simulink model "PRBS_Test"  (R2019a)
settings: Solver=FixedStepAuto  StartTime=0.0  StopTime=TSim  FixedStep=0.2  RelTol=1e-3
values from neighbouring files (symbols this model uses):
  AMtx = [-8.08083e-02, -1.00674e-01, -1.60269e-01, -2.19865e-01, -2.79461e-01, -3.39057e-01, -3.98653e-01, -4.58249e-01, -5.17844e-01, -5.77440e-01, -6.37036e-01, -6.96632e-01]    [Test.m]
  BMtx = [1.54238e+05, 1.56531e+05, 1.63413e+05, 1.70294e+05, 1.77175e+05, 1.84056e+05, 1.90937e+05, 1.97818e+05, 2.04700e+05, 2.11581e+05, 2.18462e+05, 2.25343e+05]    [Test.m]
  NCMtx = ones(1,length(AMtx))    [Test.m]
  NDMtx = 0 * ones(1,length(AMtx))    [Test.m]
  NMtx = 23042*[2.16995e-02, 4.33990e-02, 1.08498e-01, 1.73596e-01, 2.38695e-01, 3.03793e-01, 3.68892e-01, 4.33990e-01, 4.99089e-01, 5.64187e-01, 6.29286e-01, 6.94384e-01]    [Test.m]
  Num_Switch = 50    [MissionBlocks.m]    (also in Test.m = 1)
  Percent = 0.1    [MissionBlocks.m]    (also in Test.m)
  RPM = NMtx(2)    [Test.m]
  Samp_end = 2    [MissionBlocks.m]    (also in Test.m)
  Samp_start = 100    [MissionBlocks.m]    (also in Test.m)
  Samp_Switch = 2    [MissionBlocks.m]    (also in Test.m = 1000)
  Ts = 0.2    [MissionBlocks.m]    (also in Test.m)
  Wf = [0.01335 0.01669 0.02 0.025 0.03 0.0334 0.04172 0.05 0.05841 0.06676]    [MissionBlocks.m]    (also in Test.m = WfMtx(2))
  WfMtx = [3.35319e-03, 4.47091e-03, 7.87431e-03, 1.14579e-02, 1.66929e-02, 2.16627e-02, 2.55503e-02, 2.86499e-02, 3.21360e-02, 3.58686e-02, 4.06799e-02, 4.63335e-02]    [Test.m]
libraries: ctrlSharedLib x2
settings Model: Creator=anton  LastModifiedBy=anton

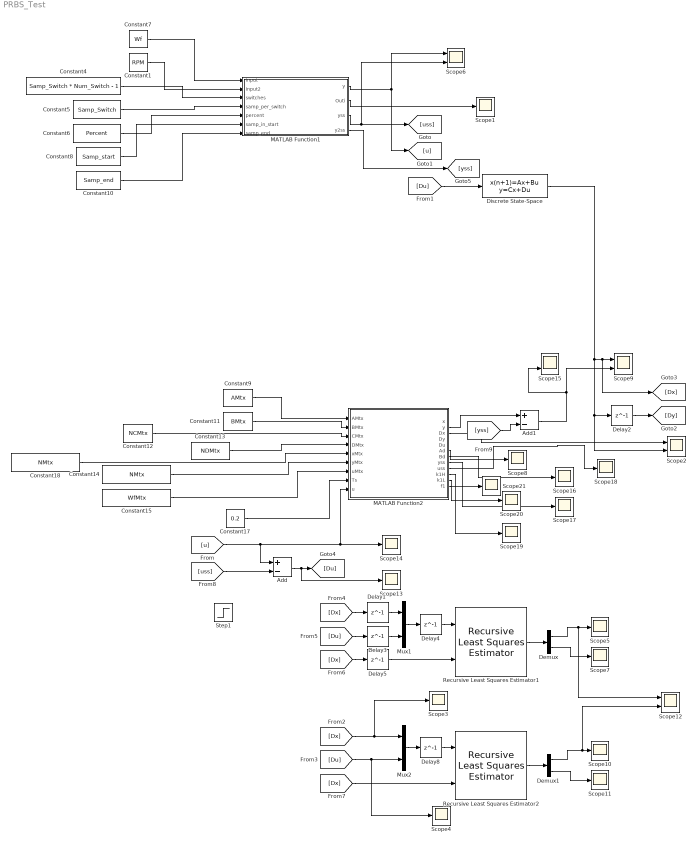
== system PRBS_Test ==
  Add : Sum  Inputs=+-
  Add1 : Sum  Inputs=+-
  Constant1 : Constant  Value=RPM
  Constant10 : Constant  Value=Samp_end
  Constant11 : Constant  Value=BMtx
  Constant12 : Constant  Value=NCMtx
  Constant13 : Constant  Value=NDMtx
  Constant14 : Constant  Value=NMtx
  Constant15 : Constant  Value=WfMtx
  Constant17 : Constant  Value=0.2
  Constant18 : Constant  Value=NMtx
  Constant4 : Constant  Value=Samp_Switch * Num_Switch - 1
  Constant5 : Constant  Value=Samp_Switch
  Constant6 : Constant  Value=Percent
  Constant7 : Constant  Value=Wf
  Constant8 : Constant  Value=Samp_start
  Constant9 : Constant  Value=AMtx
  Delay{1..5,8} (6 alike) : Delay  DelayLength=1  SampleTime=Ts
  Demux : Demux  Outputs=2
  Demux1 : Demux  Outputs=2
  Discrete State-Space : DiscreteStateSpace  A=0.9801  B=3.099e04  D=0  SampleTime=0.2
  MATLAB Function1 : MATLAB Function  TreatAsAtomicUnit=on
  MATLAB Function2 : MATLAB Function  TreatAsAtomicUnit=on
  Mux1 : Mux  Inputs=2
  Mux2 : Mux  Inputs=2
  Recursive Least Squares Estimator1 : ctrlSharedLib/Recursive Least Squares Estimator  InitialEstimateSource=None  InitialParameterData=2  P0=1e4  InitialRegressors=0  InitialOutputs=0  History=Infinite  WindowLength=200  EstimationMethod=Forgetting Factor  AdaptationParameter=0.5  HasTimeVaryingAdaptationParameter=off  NormalizationBias=eps  OutputError=off  OutputP=off  AddEnablePort=off  InputProcessing=Sample-based  Ts=Ts
      settings: SourceProductName=Control System Toolbox  SourceProductBaseCode=CT
  Recursive Least Squares Estimator2 : ctrlSharedLib/Recursive Least Squares Estimator  InitialEstimateSource=None  InitialParameterData=2  P0=1e4  InitialRegressors=0  InitialOutputs=0  History=Infinite  WindowLength=200  EstimationMethod=Forgetting Factor  AdaptationParameter=0.5  HasTimeVaryingAdaptationParameter=off  NormalizationBias=eps  OutputError=off  OutputP=off  AddEnablePort=off  InputProcessing=Sample-based  Ts=Ts
      settings: SourceProductName=Control System Toolbox  SourceProductBaseCode=CT
  Scope{1,3..5,7..8,10..11,13..14,16..21} (16 alike) : Scope
  Scope{2,6,9,12,15} (5 alike) : Scope  NumInputPorts=2
  Step1 : Step  Time=50  Before=1.5  After=2.7  SampleTime=0
  wires:
  Constant6/1 -> MATLAB Function1/5(percent)
  Constant5/1 -> MATLAB Function1/4(samp_per_switch)
  Constant4/1 -> MATLAB Function1/3(switches)
  MATLAB Function1/1(y) -> Scope6/1, [u]
  Constant7/1 -> MATLAB Function1/1(Input)
  Constant8/1 -> MATLAB Function1/6(samp_in_start)
  Constant10/1 -> MATLAB Function1/7(samp_end)
  Constant9/1 -> MATLAB Function2/1(AMtx)
  Constant11/1 -> MATLAB Function2/2(BMtx)
  Constant12/1 -> MATLAB Function2/3(CMtx)
  Constant13/1 -> MATLAB Function2/4(DMtx)
  Constant14/1 -> MATLAB Function2/6(yMtx)
  Constant15/1 -> MATLAB Function2/7(uMtx)
  [u] -> Add/1, Scope14/1, MATLAB Function2/9(u)
  Constant17/1 -> MATLAB Function2/8(Ts)
  Constant18/1 -> MATLAB Function2/5(xMtx)
  MATLAB Function2/3(Dx) -> Scope2/1
  Recursive Least Squares Estimator1/1 -> Demux/1
  Demux/1 -> Scope12/1, Scope5/1
  Demux/2 -> Scope7/1
  Mux1/1 -> Delay4/1
  [Dx] -> Delay1/1
  [Du] -> Delay3/1
  [Dx] -> Delay5/1
  MATLAB Function2/2(y) -> Add1/1
  [Du] -> Discrete State-Space/1
  MATLAB Function1/2(Outi) -> Scope1/1
  Delay1/1 -> Mux1/1
  Delay3/1 -> Mux1/2
  Delay4/1 -> Recursive Least Squares Estimator1/1
  Delay5/1 -> Recursive Least Squares Estimator1/2
  Delay2/1 -> [Dy]
  Discrete State-Space/1 -> Scope2/2, Delay2/1, [Dx], Scope9/1
  [Dx] -> Recursive Least Squares Estimator2/2
  Delay8/1 -> Recursive Least Squares Estimator2/1
  [Du] -> Scope4/1, Mux2/2
  [Dx] -> Scope3/1, Mux2/1
  Mux2/1 -> Delay8/1
  Demux1/2 -> Scope11/1
  Demux1/1 -> Scope12/2, Scope10/1
  Recursive Least Squares Estimator2/1 -> Demux1/1
  MATLAB Function1/3(yss) -> Scope6/2, [uss]
  Add/1 -> Scope13/1, [Du]
  [uss] -> Add/2
  Constant1/1 -> MATLAB Function1/2(Input2)
  MATLAB Function1/4(y2ss) -> [yss]
  [yss] -> Add1/2
  Add1/1 -> Scope15/2, Scope9/2
  MATLAB Function2/6(Ad) -> Scope8/1
  MATLAB Function2/7(Bd) -> Scope16/1
  MATLAB Function2/8(yss) -> Scope17/1
  MATLAB Function2/9(uss) -> Scope18/1
  MATLAB Function2/10(k1H) -> Scope19/1
  MATLAB Function2/11(k1L) -> Scope20/1
  MATLAB Function2/12(f1) -> Scope21/1

== matlab function PRBS_Test/MATLAB Function1 ==
  settings: updateMethod=DISCRETE  sampleTime=0.2
  data: Input input; Input2 input; y output; switches input; samp_per_switch input; percent input; samp_in_start input; samp_end input; Outi output; yss output; y2ss output
function [y,Outi,yss,y2ss] = fcn(Input,Input2,switches,samp_per_switch,percent,samp_in_start,samp_end)
     
persistent state;
persistent u;
persistent switch_count;
persistent switch_stay;
persistent level_count;
persistent output

persistent i;

%Initiates outputs
y = Input(1);
y2ss = Input2(1);
yss = Input(1);
LengIn = length(Input);
Outi = 0;

%Initiates persistent variables
if isempty(state)

    state = 0;
    switch_count = 0;
    switch_stay = 0;
    level_count = 1;
    output = Input(1);
    u = Input(1);
    i = 0;

    return;

end

switch state
    case 0
        %Updates output
        output = u;
        yss = u;
        y2ss = Input2(level_count);
        %Updates the number of samples of signal holding
        switch_stay = switch_stay + 1;
        %Verifies if signal has been held for enought sample periods
        if switch_stay == samp_in_start
            state = 1;
            switch_stay = samp_per_switch;
        end
    case 1
        %Verifies if signal has been held for enought sample periods
        if switch_stay == samp_per_switch && switch_count <= switches
            %Generates a random numver for coefficient generation
            coeff = rand(1,1);
            %Determines the coefficient for oscilation around input value
            if coeff > 0.5
                coeff = 1;
            else
                coeff = -1;
            end
            %Updates output
            output = u * (1 + coeff * percent);
            switch_stay = 0;
            i = i+1;
        end
        
        %Updates switch count
        switch_stay = switch_stay + 1;
        switch_count = switch_count + 1;
        
        %All switches have been accomplisehd
        if switch_count > switches
            state = 2;
            switch_stay = 0;
            switch_count = 0;
            i = 0;
        end
        
    case 2
        %If number of switches have been reached, the output must remain
        %equal current input level
        output = u;
        %Updates switch count
        switch_stay = switch_stay + 1;
        %If output is at current lavel for enough samples, next state is
        %activated
        if switch_stay >= samp_end
            state = 3;
            switch_stay = 0;
        end
        %If change is deteced, cycle starts again
    case 3
        %Updates signal level counter
        level_count = level_count + 1;
        %Updates u for next input level if possible
        if level_count <= LengIn
            u = Input(level_count);
            y2ss = Input2(level_count);
            state = 0;
        end
        
end

%Updates fuel level for mission
y = output;
%Updates i - shows how many times the output is calculated while in prbs
Outi = i;

== matlab function PRBS_Test/MATLAB Function2 ==
  settings: updateMethod=DISCRETE  sampleTime=0.2
  data: x output; AMtx input; y output; BMtx input; CMtx input; DMtx input; xMtx input; yMtx input; uMtx input; Ts input; u input; Dx output; Dy output; Du output; Ad output; Bd output; yss output; uss output; k1H output; k1L output; f1 output
function [x,y,Dx,Dy,Du,Ad,Bd,yss,uss,k1H,k1L,f1] = fcn(AMtx,BMtx,CMtx,DMtx,xMtx,yMtx,uMtx,Ts,u)
     
AMtx = AMtx';
BMtx = BMtx';
CMtx = CMtx';
DMtx = DMtx';
yMtx = yMtx';
xMtx = xMtx';
uMtx = uMtx';



persistent xIn
persistent yIn
persistent ICCalc

y = 0;
yss = 0;
x = 0;
xss = 0;
uss = 0;
A = 0;
B = 0;
C = 0;
D = 0;
Dx = 0;
Dy = 0;
Du = 0;

Ad = 0;
Bd = 0;
xss = 0;
uss = 0;

k1H = 0;
k1L = 0;
f1 = 0;

%Initiates persistent variables
if isempty(yIn)

    yIn = 0;
    xIn = 0;
    ICCalc = 0;
    
    return;

end

%Calculation of initial conditions
if ICCalc == 0
    %Updates ICCalc with 1
    ICCalc = 1;
    %Calculates index using u and uMtx for finding initial y
    [k1H,k1L,f1,k2H,k2L,f2,k3H,k3L,f3] = Lookup3d(0,0,uMtx,0,0,u);
    yIn = LookupValue(k1H,k1L,f1,k2H,k2L,f2,k3H,k3L,f3,yMtx);
    xIn = LookupValue(k1H,k1L,f1,k2H,k2L,f2,k3H,k3L,f3,xMtx);
    
    return
    
end

if ICCalc == 1
    [k1H,k1L,f1,k2H,k2L,f2,k3H,k3L,f3] = Lookup3d(0,0,yMtx,0,0,yIn);
    A = LookupValue(k1H,k1L,f1,k2H,k2L,f2,k3H,k3L,f3,AMtx);
    B = LookupValue(k1H,k1L,f1,k2H,k2L,f2,k3H,k3L,f3,BMtx);
    C = LookupValue(k1H,k1L,f1,k2H,k2L,f2,k3H,k3L,f3,CMtx);
    D = LookupValue(k1H,k1L,f1,k2H,k2L,f2,k3H,k3L,f3,DMtx);
    uss = LookupValue(k1H,k1L,f1,k2H,k2L,f2,k3H,k3L,f3,uMtx);
    xss = LookupValue(k1H,k1L,f1,k2H,k2L,f2,k3H,k3L,f3,xMtx);
    yss = LookupValue(k1H,k1L,f1,k2H,k2L,f2,k3H,k3L,f3,yMtx);
end

%Calculates digital state-space for current model
Ad = exp(A * Ts);
Bd = (exp(A * Ts) - 1)*B/A;
Cd = C;
Dd = D;

%Updates the output with current value of xIn (yIn must be delayed by one
%sample from xIn)
yIn = yss + Cd * (xIn-xss) + Dd * (u-uss);
%Updates the state value
xIn = xss +  Ad * (xIn-xss) + Bd * (u-uss);


%Updates fuel level for mission
x = xIn;
Dx = xIn - xss;
y = yIn;
Dy = yIn - yss;
Du = u - uss;

%Updates xIn
% xIn = xk1;
